simulink model "Slx003_MHMP"  (R2017b)
settings: Solver=VariableStepAuto  StartTime=0.0  StopTime=50  RelTol=1e-3
values from neighbouring files (symbols this model uses):
  Nbar = rscale(sys_ss, K_lqr)    [Cmd002_ChonPoleTinhK_MHMP.m]
libraries: slident x1
settings Model: Creator=Dell  LastModifiedBy=Dell

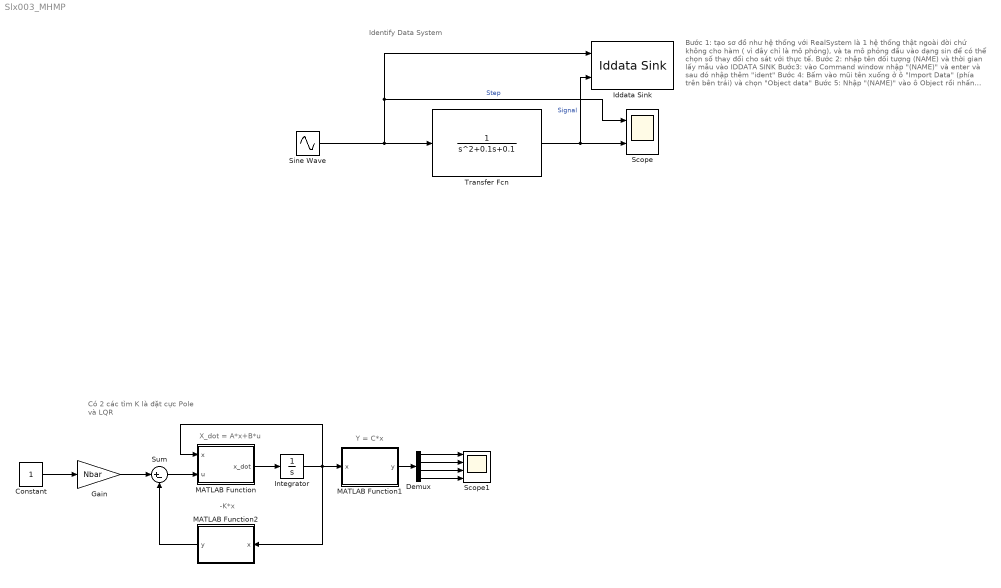
== system Slx003_MHMP ==
  note: Bước 1: tạo sơ đồ như hệ thống với RealSystem là 1 hệ thống thật ngoài đời chứ không cho hàm ( vì đây chỉ là mô phỏng), và ta mô phỏng đầu vào dạng sin để có thể chọn số thay đổi cho sát với thực tế.
      |
      | Bước 2: nhập tên đối tượng (NAME) và thời gian lấy mẫu vào IDDATA SINK
      |
      | Bước3: vào Command window nhập "(NAME)" và enter và sau đó nhập thêm "ident"
      |
      | Bước 4: Bấm vào mũi tên xuống ở ô "Import Data" (phía trên bên trái) và chọn "Object data"
      |
      |  Bước 5: Nhập "(NAME)" vào ô Object rồi nhấn "enter" xong nhấn vào ô "Import" rồi chọn "Close"
      |
      |  Bước 6: (Ở bảng bước 4): (có thể bấm tick vào "Time Plot" để xem dạng đồ thị ngõ vào và ra) Bấm chọn mũi tên xuống ở "Estimate" (ở giữa hơi lệch bên trái dưới) chọn "Transfer Function..." rồi nhập những thứ cần thiết rồi chọn "Continuous" (liên tục) hoặc "Discrete" (rời rạc) xong bấm "Estimate" và đợi chạy xong.
      |
      | Bước 7:(quay lại bảng bước 4): Chọn double click vào ô bên phải để xem hàm truyền
  note: Identify Data System
  note: Có 2 các tìm K là đặt cực Pole và LQR
  note: Y = C*x
  note: -K*x
  note: X_dot = A*x+B*u
  Constant : Constant
  Demux : Demux
  Gain : Gain  Gain=Nbar
  Iddata Sink : slident/Iddata Sink  datasetname=Test  Ts=0.1  isu=off  isy=off
      settings: SourceProductName=System Identification Toolbox  SourceProductBaseCode=ID
  Integrator : Integrator  InitialCondition=[1; -1; 2; 1]
  MATLAB Function : MATLAB Function  TreatAsAtomicUnit=on
  MATLAB Function1 : MATLAB Function  TreatAsAtomicUnit=on
  MATLAB Function2 : MATLAB Function  TreatAsAtomicUnit=on
  Scope : Scope  NumInputPorts=2
  Scope1 : Scope  NumInputPorts=4
  Sine Wave : Sin  SampleTime=0
  Sum : Sum  Inputs=|+-
  Transfer Fcn : TransferFcn  Denominator=[1 0.1 0.1]
  wires:
  Transfer Fcn/1 -> Iddata Sink/2, Scope/2  "Signal"
  Sine Wave/1 -> Transfer Fcn/1, Iddata Sink/1, Scope/1  "Step"
  MATLAB Function/1(x_dot) -> Integrator/1
  Integrator/1 -> MATLAB Function2/1(x), MATLAB Function/1(x), MATLAB Function1/1(x)
  Sum/1 -> MATLAB Function/2(u)
  MATLAB Function2/1(y) -> Sum/2
  Demux/3 -> Scope1/3
  MATLAB Function1/1(y) -> Demux/1
  Demux/2 -> Scope1/2
  Demux/1 -> Scope1/1
  Demux/4 -> Scope1/4
  Gain/1 -> Sum/1
  Constant/1 -> Gain/1

== matlab function Slx003_MHMP/MATLAB Function1 ==
  data: x input; y output
function y = fcn(x)
C = [1 0 0 0;
     0 1 0 0;
     0 0 1 0;
     0 0 0 1];
D = 0;
y = C*x + D;

== matlab function Slx003_MHMP/MATLAB Function ==
  data: x input; u input; x_dot output
function x_dot = fcn(x, u)
K1=5; K2=7; D1=40; D2=30; M1=2; M2=3;

A = [0 1 0 0;
    -K2/M2 -D2/M2 K1/M2 D1/M2;
    0 0 0 1
    (K1-K2)/M1 (D1-D2)/M1 -K1/M1 -D1/M1];

B = [0; 0; 0; 1/M1];
x_dot = A*x + B*u;

== matlab function Slx003_MHMP/MATLAB Function2 ==
  data: x input; y output
function y = fcn(x)
K = [0.0302    0.0284    0.0948    0.0362];


y = -K*x;
